simulink model "Dion_CBC_Simulink"  (R2023a)
settings: Solver=ode5  StartTime=0.0  StopTime=Inf  FixedStep=0.001  RelTol=1e-3
PostLoadFcn:
  | , if any(exist('dsrtsu_mdlpostloadfcn', 'file') ~= 0), dsrtsu_mdlpostloadfcn('Execute', bdroot); end,
InitFcn:
  | , if any(exist('rtifpga_mdlclblib', 'file') ~= 0), rtifpga_mdlclblib('Init', bdroot); end,
values from neighbouring files (symbols this model uses):
  k_harmonics = 7    [freq_sweep_continous.m]
libraries: simulink x3, rti1202lib_adc_class1 x3, rti1202lib_dac_class1 x1, rti1202lib_base x1
(part 2 of 2)

== system Dion_CBC_Simulink/invasiveness_estimator/get secondary ==
  Vector : Inport
  Demux : Demux  Outputs=[1, 1, k_harmonics-1, 1, k_harmonics-1]
  Mux : Mux  Inputs=2
  Terminator1 : Terminator
  Terminator2 : Terminator
  Terminator3 : Terminator
  secondary : Outport
  wires:
  Demux/1 -> Terminator2/1
  Mux/1 -> secondary/1
  Demux/3 -> Mux/1
  Demux/5 -> Mux/2
  Vector/1 -> Demux/1
  Demux/2 -> Terminator1/1
  Demux/4 -> Terminator3/1

== system Dion_CBC_Simulink/sig_reconstructor/Harmonic Basis Gen1 ==
  fund_freq : Inport
  Cos : Trigonometry  Operator=cos
  DC : Constant
  Gain1 : Gain  Gain=2*pi
  Integrator : Integrator
  Mux : Mux  Inputs=3
  Product : Product
  Sin : Trigonometry
  harmonics_array : Constant  Value=1:k_harmonics
  harmonic_basis : Outport  OutDataTypeStr=double  SampleTime=0
  wires:
  Gain1/1 -> Sin/1, Cos/1
  Mux/1 -> harmonic_basis/1
  Integrator/1 -> Product/1
  Cos/1 -> Mux/2
  Product/1 -> Gain1/1
  Sin/1 -> Mux/3
  harmonics_array/1 -> Product/2
  fund_freq/1 -> Integrator/1
  DC/1 -> Mux/1

== system Dion_CBC_Simulink/x_reconstructor/Harmonic Basis Gen1 ==
  fund_freq : Inport
  Cos : Trigonometry  Operator=cos
  DC : Constant
  Gain1 : Gain  Gain=2*pi
  Integrator : Integrator
  Mux : Mux  Inputs=3
  Product : Product
  Sin : Trigonometry
  harmonics_array : Constant  Value=1:k_harmonics
  harmonic_basis : Outport  OutDataTypeStr=double  SampleTime=0
  wires:
  Gain1/1 -> Sin/1, Cos/1
  Mux/1 -> harmonic_basis/1
  Integrator/1 -> Product/1
  Cos/1 -> Mux/2
  Product/1 -> Gain1/1
  Sin/1 -> Mux/3
  harmonics_array/1 -> Product/2
  fund_freq/1 -> Integrator/1
  DC/1 -> Mux/1

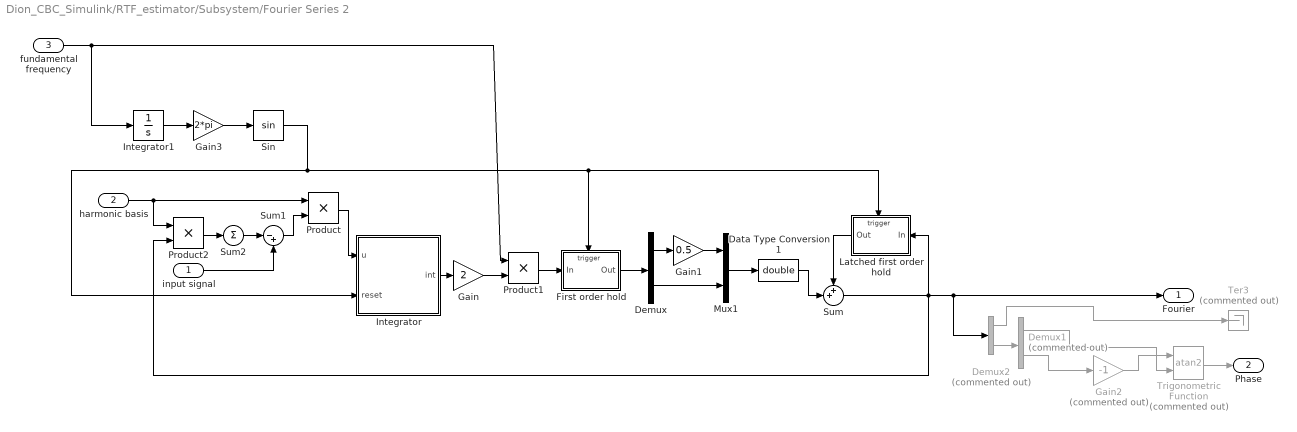
== system Dion_CBC_Simulink/RTF_estimator/Subsystem/Fourier Series 2 ==
  input signal : Inport
  harmonic basis : Inport  Port=2
  fundamental frequency : Inport  Port=3
  Data Type Conversion1 : DataTypeConversion  OutDataTypeStr=double  SaturateOnIntegerOverflow=off  RndMeth=Floor
  Demux : Demux  Outputs=[1 -1]
  Demux1 : Demux  Commented=on  Outputs=2
  Demux2 : Demux  Commented=on  Outputs=[1 -1]
  First order hold : Subsystem  TreatAsAtomicUnit=on
  Gain : Gain  Gain=2
  Gain1 : Gain  Gain=0.5
  Gain2 : Gain  Commented=on  Gain=-1
  Gain3 : Gain  Gain=2*pi
  Integrator : Subsystem
  Integrator1 : Integrator
  Latched first order hold : Subsystem  TreatAsAtomicUnit=on
  Mux1 : Mux  Inputs=2
  Product : Product  RndMeth=Zero
  Product1 : Product  RndMeth=Zero
  Product2 : Product  RndMeth=Zero
  Sin : Trigonometry
  Sum : Sum  Tag=Test  Inputs=++|
  Sum1 : Sum  Inputs=|-+
  Sum2 : Sum  Inputs=|+|
  Ter3 : Terminator  Commented=on
  Trigonometric Function : Trigonometry  Commented=on  Operator=atan2
  Fourier : Outport
  Phase : Outport  Port=2
  wires:
  fundamental frequency/1 -> Product1/1, Integrator1/1
  Integrator1/1 -> Gain3/1
  Gain3/1 -> Sin/1
  Demux2/1 -> Ter3/1
  Demux2/2 -> Demux1/1
  Gain2/1 -> Trigonometric Function/1
  Demux1/2 -> Gain2/1
  Demux1/1 -> Trigonometric Function/2
  Product/1 -> Integrator/1(u)
  Trigonometric Function/1 -> Phase/1
  Sum2/1 -> Sum1/1
  harmonic basis/1 -> Product2/1, Product/1
  input signal/1 -> Sum1/2
  Product2/1 -> Sum2/1
  Sum1/1 -> Product/2
  Latched first order hold/1(Out) -> Sum/1
  Sum/1 -> Demux2/1, Fourier/1, Latched first order hold/1(In), Product2/2
  Data Type Conversion1/1 -> Sum/2
  Mux1/1 -> Data Type Conversion1/1
  First order hold/1(Out) -> Demux/1
  Demux/2 -> Mux1/2
  Gain1/1 -> Mux1/1
  Demux/1 -> Gain1/1
  Integrator/1(int) -> Gain/1
  Sin/1 -> Latched first order hold/Trigger, First order hold/Trigger, Integrator/2(reset)
  Gain/1 -> Product1/2
  Product1/1 -> First order hold/1(In)

== system Dion_CBC_Simulink/RTF_estimator/Subsystem/Harmonic Basis Gen1 ==
  fund_freq : Inport
  Cos : Trigonometry  Operator=cos
  DC : Constant
  Gain1 : Gain  Gain=2*pi
  Integrator : Integrator
  Mux : Mux  Inputs=3
  Product : Product
  Sin : Trigonometry
  harmonics_array : Constant  Value=1:k_harmonics
  harmonic_basis : Outport  OutDataTypeStr=double  SampleTime=0
  wires:
  Gain1/1 -> Sin/1, Cos/1
  Mux/1 -> harmonic_basis/1
  Integrator/1 -> Product/1
  Cos/1 -> Mux/2
  Product/1 -> Gain1/1
  Sin/1 -> Mux/3
  harmonics_array/1 -> Product/2
  fund_freq/1 -> Integrator/1
  DC/1 -> Mux/1

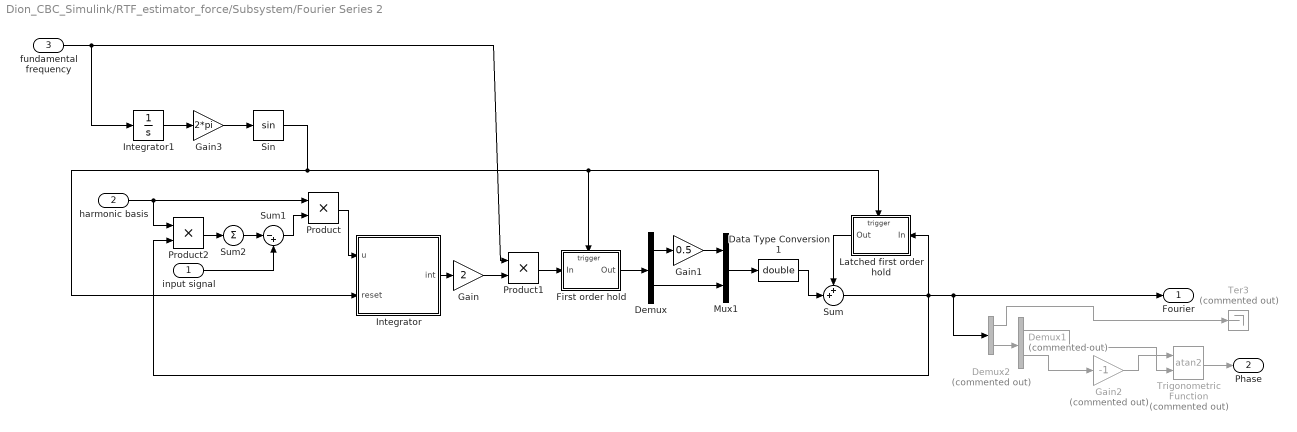
== system Dion_CBC_Simulink/RTF_estimator_force/Subsystem/Fourier Series 2 ==
  input signal : Inport
  harmonic basis : Inport  Port=2
  fundamental frequency : Inport  Port=3
  Data Type Conversion1 : DataTypeConversion  OutDataTypeStr=double  SaturateOnIntegerOverflow=off  RndMeth=Floor
  Demux : Demux  Outputs=[1 -1]
  Demux1 : Demux  Commented=on  Outputs=2
  Demux2 : Demux  Commented=on  Outputs=[1 -1]
  First order hold : Subsystem  TreatAsAtomicUnit=on
  Gain : Gain  Gain=2
  Gain1 : Gain  Gain=0.5
  Gain2 : Gain  Commented=on  Gain=-1
  Gain3 : Gain  Gain=2*pi
  Integrator : Subsystem
  Integrator1 : Integrator
  Latched first order hold : Subsystem  TreatAsAtomicUnit=on
  Mux1 : Mux  Inputs=2
  Product : Product  RndMeth=Zero
  Product1 : Product  RndMeth=Zero
  Product2 : Product  RndMeth=Zero
  Sin : Trigonometry
  Sum : Sum  Tag=Test  Inputs=++|
  Sum1 : Sum  Inputs=|-+
  Sum2 : Sum  Inputs=|+|
  Ter3 : Terminator  Commented=on
  Trigonometric Function : Trigonometry  Commented=on  Operator=atan2
  Fourier : Outport
  Phase : Outport  Port=2
  wires:
  Product1/1 -> First order hold/1(In)
  Gain/1 -> Product1/2
  Sin/1 -> Integrator/2(reset), First order hold/Trigger, Latched first order hold/Trigger
  Integrator/1(int) -> Gain/1
  Demux/1 -> Gain1/1
  Gain1/1 -> Mux1/1
  Demux/2 -> Mux1/2
  First order hold/1(Out) -> Demux/1
  Mux1/1 -> Data Type Conversion1/1
  Data Type Conversion1/1 -> Sum/2
  Sum/1 -> Product2/2, Latched first order hold/1(In), Fourier/1, Demux2/1
  Latched first order hold/1(Out) -> Sum/1
  Sum1/1 -> Product/2
  Product2/1 -> Sum2/1
  input signal/1 -> Sum1/2
  harmonic basis/1 -> Product/1, Product2/1
  Sum2/1 -> Sum1/1
  Trigonometric Function/1 -> Phase/1
  Product/1 -> Integrator/1(u)
  Demux1/1 -> Trigonometric Function/2
  Demux1/2 -> Gain2/1
  Gain2/1 -> Trigonometric Function/1
  Demux2/2 -> Demux1/1
  Demux2/1 -> Ter3/1
  Gain3/1 -> Sin/1
  Integrator1/1 -> Gain3/1
  fundamental frequency/1 -> Integrator1/1, Product1/1

== system Dion_CBC_Simulink/RTF_estimator_force/Subsystem/Harmonic Basis Gen1 ==
  fund_freq : Inport
  Cos : Trigonometry  Operator=cos
  DC : Constant
  Gain1 : Gain  Gain=2*pi
  Integrator : Integrator
  Mux : Mux  Inputs=3
  Product : Product
  Sin : Trigonometry
  harmonics_array : Constant  Value=1:k_harmonics
  harmonic_basis : Outport  OutDataTypeStr=double  SampleTime=0
  wires:
  DC/1 -> Mux/1
  fund_freq/1 -> Integrator/1
  harmonics_array/1 -> Product/2
  Sin/1 -> Mux/3
  Product/1 -> Gain1/1
  Cos/1 -> Mux/2
  Integrator/1 -> Product/1
  Mux/1 -> harmonic_basis/1
  Gain1/1 -> Cos/1, Sin/1

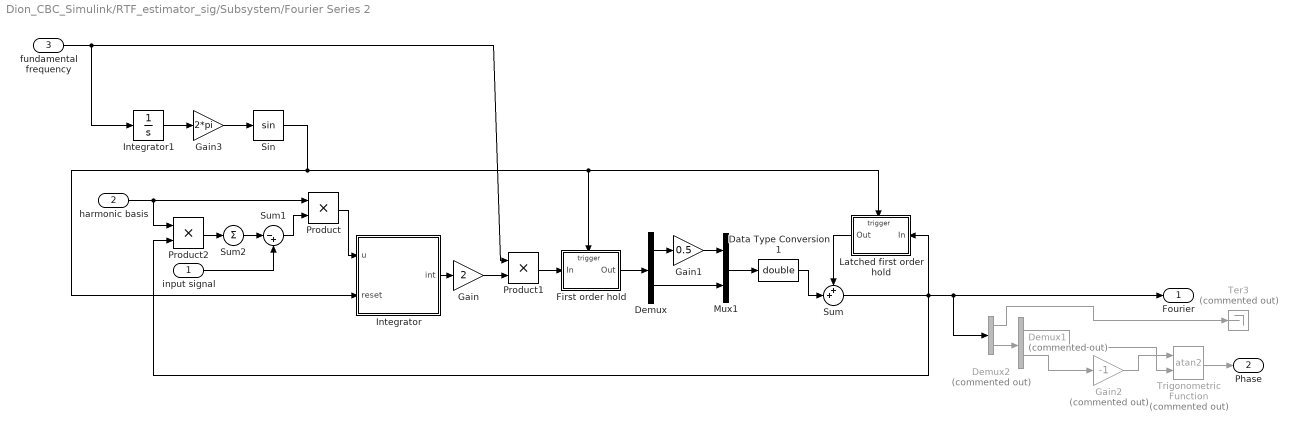
== system Dion_CBC_Simulink/RTF_estimator_sig/Subsystem/Fourier Series 2 ==
  input signal : Inport
  harmonic basis : Inport  Port=2
  fundamental frequency : Inport  Port=3
  Data Type Conversion1 : DataTypeConversion  OutDataTypeStr=double  SaturateOnIntegerOverflow=off  RndMeth=Floor
  Demux : Demux  Outputs=[1 -1]
  Demux1 : Demux  Commented=on  Outputs=2
  Demux2 : Demux  Commented=on  Outputs=[1 -1]
  First order hold : Subsystem  TreatAsAtomicUnit=on
  Gain : Gain  Gain=2
  Gain1 : Gain  Gain=0.5
  Gain2 : Gain  Commented=on  Gain=-1
  Gain3 : Gain  Gain=2*pi
  Integrator : Subsystem
  Integrator1 : Integrator
  Latched first order hold : Subsystem  TreatAsAtomicUnit=on
  Mux1 : Mux  Inputs=2
  Product : Product  RndMeth=Zero
  Product1 : Product  RndMeth=Zero
  Product2 : Product  RndMeth=Zero
  Sin : Trigonometry
  Sum : Sum  Tag=Test  Inputs=++|
  Sum1 : Sum  Inputs=|-+
  Sum2 : Sum  Inputs=|+|
  Ter3 : Terminator  Commented=on
  Trigonometric Function : Trigonometry  Commented=on  Operator=atan2
  Fourier : Outport
  Phase : Outport  Port=2
  wires:
  fundamental frequency/1 -> Product1/1, Integrator1/1
  Integrator1/1 -> Gain3/1
  Gain3/1 -> Sin/1
  Demux2/1 -> Ter3/1
  Demux2/2 -> Demux1/1
  Gain2/1 -> Trigonometric Function/1
  Demux1/2 -> Gain2/1
  Demux1/1 -> Trigonometric Function/2
  Product/1 -> Integrator/1(u)
  Trigonometric Function/1 -> Phase/1
  Sum2/1 -> Sum1/1
  harmonic basis/1 -> Product2/1, Product/1
  input signal/1 -> Sum1/2
  Product2/1 -> Sum2/1
  Sum1/1 -> Product/2
  Latched first order hold/1(Out) -> Sum/1
  Sum/1 -> Demux2/1, Fourier/1, Latched first order hold/1(In), Product2/2
  Data Type Conversion1/1 -> Sum/2
  Mux1/1 -> Data Type Conversion1/1
  First order hold/1(Out) -> Demux/1
  Demux/2 -> Mux1/2
  Gain1/1 -> Mux1/1
  Demux/1 -> Gain1/1
  Integrator/1(int) -> Gain/1
  Sin/1 -> Latched first order hold/Trigger, First order hold/Trigger, Integrator/2(reset)
  Gain/1 -> Product1/2
  Product1/1 -> First order hold/1(In)

== system Dion_CBC_Simulink/RTF_estimator_sig/Subsystem/Harmonic Basis Gen1 ==
  fund_freq : Inport
  Cos : Trigonometry  Operator=cos
  DC : Constant
  Gain1 : Gain  Gain=2*pi
  Integrator : Integrator
  Mux : Mux  Inputs=3
  Product : Product
  Sin : Trigonometry
  harmonics_array : Constant  Value=1:k_harmonics
  harmonic_basis : Outport  OutDataTypeStr=double  SampleTime=0
  wires:
  Gain1/1 -> Sin/1, Cos/1
  Mux/1 -> harmonic_basis/1
  Integrator/1 -> Product/1
  Cos/1 -> Mux/2
  Product/1 -> Gain1/1
  Sin/1 -> Mux/3
  harmonics_array/1 -> Product/2
  fund_freq/1 -> Integrator/1
  DC/1 -> Mux/1

== system Dion_CBC_Simulink/RTI Data/RTI Data Store/RTI Data Store ==
  RTI Data Store : Subsystem  mask(RTI_DATA_STORE){}
      mask help:
      | RTI Data Store Block. This block is used by RTI to store internal model dependent data. Deleting this block will result in data loss.
      |
      | NEVER DELETE, COPY, OR MODIFY THIS BLOCK!
      mask Help:
      | RTI Data Store Block. This block is used by RTI to store internal model dependent data. Deleting this block will result in data loss.
      | 
      | NEVER DELETE, COPY, OR MODIFY THIS BLOCK!
      mask Display: text(0.5, 0.5, ' ', 'HorizontalAlignment', 'center');

== system Dion_CBC_Simulink/RTF_estimator/Subsystem/Fourier Series 2/First order hold ==
  In : Inport  LatchByDelayingOutsideSignal=on
  Trigger : TriggerPort  VariantControl=(inherit)
  Out : Outport
  wires:
  In/1 -> Out/1

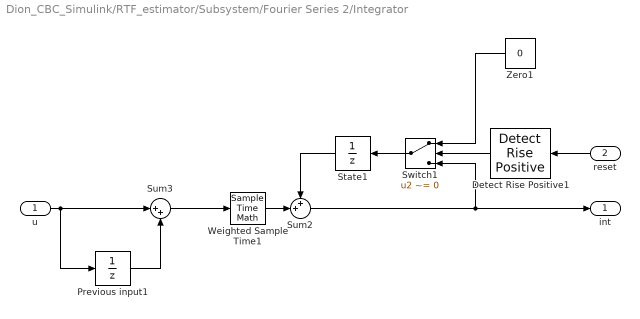
== system Dion_CBC_Simulink/RTF_estimator/Subsystem/Fourier Series 2/Integrator ==
  u : Inport
  reset : Inport  Port=2
  Detect Rise Positive1 : simulink/Logic and Bit Operations/Detect Rise Positive  vinit=0  OutDataTypeStr=uint8
  Previous input1 : UnitDelay  SampleTime=-1  HasFrameUpgradeWarning=on
  State1 : UnitDelay  SampleTime=-1  HasFrameUpgradeWarning=on
  Sum2 : Sum  Inputs=++|
  Sum3 : Sum  Inputs=|++
  Switch1 : Switch  Criteria=u2 ~= 0  SaturateOnIntegerOverflow=off  InputSameDT=off
  Weighted Sample Time1 : SampleTimeMath  TsampMathOp=*  weightValue=0.5
  Zero1 : Constant  Value=0
  int : Outport
  wires:
  State1/1 -> Sum2/1
  Sum2/1 -> Switch1/3, int/1
  Weighted Sample Time1/1 -> Sum2/2
  Sum3/1 -> Weighted Sample Time1/1
  u/1 -> Sum3/1, Previous input1/1
  Previous input1/1 -> Sum3/2
  reset/1 -> Detect Rise Positive1/1
  Switch1/1 -> State1/1
  Zero1/1 -> Switch1/1
  Detect Rise Positive1/1 -> Switch1/2

== system Dion_CBC_Simulink/RTF_estimator/Subsystem/Fourier Series 2/Latched first order hold ==
  In : Inport  LatchByDelayingOutsideSignal=on
  Trigger : TriggerPort  VariantControl=(inherit)
  Out : Outport
  wires:
  In/1 -> Out/1

== system Dion_CBC_Simulink/RTF_estimator_force/Subsystem/Fourier Series 2/First order hold ==
  In : Inport  LatchByDelayingOutsideSignal=on
  Trigger : TriggerPort  VariantControl=(inherit)
  Out : Outport
  wires:
  In/1 -> Out/1

== system Dion_CBC_Simulink/RTF_estimator_force/Subsystem/Fourier Series 2/Integrator ==
  u : Inport
  reset : Inport  Port=2
  Detect Rise Positive1 : simulink/Logic and Bit Operations/Detect Rise Positive  vinit=0  OutDataTypeStr=uint8
  Previous input1 : UnitDelay  SampleTime=-1  HasFrameUpgradeWarning=on
  State1 : UnitDelay  SampleTime=-1  HasFrameUpgradeWarning=on
  Sum2 : Sum  Inputs=++|
  Sum3 : Sum  Inputs=|++
  Switch1 : Switch  Criteria=u2 ~= 0  SaturateOnIntegerOverflow=off  InputSameDT=off
  Weighted Sample Time1 : SampleTimeMath  TsampMathOp=*  weightValue=0.5
  Zero1 : Constant  Value=0
  int : Outport
  wires:
  Detect Rise Positive1/1 -> Switch1/2
  Zero1/1 -> Switch1/1
  Switch1/1 -> State1/1
  reset/1 -> Detect Rise Positive1/1
  Previous input1/1 -> Sum3/2
  u/1 -> Previous input1/1, Sum3/1
  Sum3/1 -> Weighted Sample Time1/1
  Weighted Sample Time1/1 -> Sum2/2
  Sum2/1 -> int/1, Switch1/3
  State1/1 -> Sum2/1

== system Dion_CBC_Simulink/RTF_estimator_force/Subsystem/Fourier Series 2/Latched first order hold ==
  In : Inport  LatchByDelayingOutsideSignal=on
  Trigger : TriggerPort  VariantControl=(inherit)
  Out : Outport
  wires:
  In/1 -> Out/1

== system Dion_CBC_Simulink/RTF_estimator_sig/Subsystem/Fourier Series 2/First order hold ==
  In : Inport  LatchByDelayingOutsideSignal=on
  Trigger : TriggerPort  VariantControl=(inherit)
  Out : Outport
  wires:
  In/1 -> Out/1

== system Dion_CBC_Simulink/RTF_estimator_sig/Subsystem/Fourier Series 2/Integrator ==
  u : Inport
  reset : Inport  Port=2
  Detect Rise Positive1 : simulink/Logic and Bit Operations/Detect Rise Positive  vinit=0  OutDataTypeStr=uint8
  Previous input1 : UnitDelay  SampleTime=-1  HasFrameUpgradeWarning=on
  State1 : UnitDelay  SampleTime=-1  HasFrameUpgradeWarning=on
  Sum2 : Sum  Inputs=++|
  Sum3 : Sum  Inputs=|++
  Switch1 : Switch  Criteria=u2 ~= 0  SaturateOnIntegerOverflow=off  InputSameDT=off
  Weighted Sample Time1 : SampleTimeMath  TsampMathOp=*  weightValue=0.5
  Zero1 : Constant  Value=0
  int : Outport
  wires:
  State1/1 -> Sum2/1
  Sum2/1 -> Switch1/3, int/1
  Weighted Sample Time1/1 -> Sum2/2
  Sum3/1 -> Weighted Sample Time1/1
  u/1 -> Sum3/1, Previous input1/1
  Previous input1/1 -> Sum3/2
  reset/1 -> Detect Rise Positive1/1
  Switch1/1 -> State1/1
  Zero1/1 -> Switch1/1
  Detect Rise Positive1/1 -> Switch1/2

== system Dion_CBC_Simulink/RTF_estimator_sig/Subsystem/Fourier Series 2/Latched first order hold ==
  In : Inport  LatchByDelayingOutsideSignal=on
  Trigger : TriggerPort  VariantControl=(inherit)
  Out : Outport
  wires:
  In/1 -> Out/1

== system Dion_CBC_Simulink/RTI Data/RTI Data Store/RTI Data Store/RTI Data Store ==
  RTI Data Store : Subsystem  mask(RTI_DATA_STORE){}
      mask help:
      | RTI Data Store Block. This block is used by RTI to store internal model dependent data. Deleting this block will result in data loss.
      |
      | NEVER DELETE, COPY, OR MODIFY THIS BLOCK!
      mask Help:
      | RTI Data Store Block. This block is used by RTI to store internal model dependent data. Deleting this block will result in data loss.
      | 
      | NEVER DELETE, COPY, OR MODIFY THIS BLOCK!
      mask Display: text(0.5, 0.5, ' ', 'HorizontalAlignment', 'center');

== system Dion_CBC_Simulink/RTI Data/RTI Data Store/RTI Data Store/RTI Data Store/RTI Data Store ==

== matlab function Dion_CBC_Simulink/RTF_estimator_force/MATLAB Function1 ==
  data: Coeffs input; avgCoeffs output; varCoeffs output
function [avgCoeffs, varCoeffs] = exponentialAverageWithVariance(Coeffs)
% Exponential Moving Average (EMA) and Variance (EMV) for Fourier Coefficients

% Tuning parameter
alpha = 5e-4;  % 0.001 (slow, smooth) to 0.1 (fast, responsive)

% Persistent storage
persistent avg sqAvg
if isempty(avg)
    avg = Coeffs;
    sqAvg = Coeffs.^2;
end

% EMA update
avg = alpha * Coeffs + (1 - alpha) * avg;

% EMA of square
sqAvg = alpha * (Coeffs.^2) + (1 - alpha) * sqAvg;

% Variance = E[x^2] - (E[x])^2
varCoeffs = sqAvg - avg.^2;

% Output
avgCoeffs = avg;
end

== matlab function Dion_CBC_Simulink/RTF_estimator_sig/MATLAB Function1 ==
  data: Coeffs input; avgCoeffs output; varCoeffs output
function [avgCoeffs, varCoeffs] = exponentialAverageWithVariance(Coeffs)
% Exponential Moving Average (EMA) and Variance (EMV) for Fourier Coefficients

% Tuning parameter
alpha = 5e-4;  % 0.001 (slow, smooth) to 0.1 (fast, responsive)

% Persistent storage
persistent avg sqAvg
if isempty(avg)
    avg = Coeffs;
    sqAvg = Coeffs.^2;
end

% EMA update
avg = alpha * Coeffs + (1 - alpha) * avg;

% EMA of square
sqAvg = alpha * (Coeffs.^2) + (1 - alpha) * sqAvg;

% Variance = E[x^2] - (E[x])^2
varCoeffs = sqAvg - avg.^2;

% Output
avgCoeffs = avg;
end

== matlab function Dion_CBC_Simulink/MATLAB Function1 ==
  data: Coeffs input; avgCoeffs output; varCoeffs output
function [avgCoeffs, varCoeffs] = exponentialAverageWithVariance(Coeffs)
% Exponential Moving Average (EMA) and Variance (EMV) for Fourier Coefficients

% Tuning parameter
alpha = 5e-4;  % 0.001 (slow, smooth) to 0.1 (fast, responsive)

% Persistent storage
persistent avg sqAvg
if isempty(avg)
    avg = Coeffs;
    sqAvg = Coeffs.^2;
end

% EMA update
avg = alpha * Coeffs + (1 - alpha) * avg;

% EMA of square
sqAvg = alpha * (Coeffs.^2) + (1 - alpha) * sqAvg;

% Variance = E[x^2] - (E[x])^2
varCoeffs = sqAvg - avg.^2;

% Output
avgCoeffs = avg;
end

== matlab function Dion_CBC_Simulink/Kalman_Filter/MATLAB Function ==
  data: disp_measured input; acc_measured input; q1 input; disp_estimate output; q2 input; R input; vel_estimate output
function [disp_estimate, vel_estimate] = kalman_vel_disp(disp_measured, acc_measured, q1, q2, R)
% 雙輸入雙輸出卡爾曼觀測器，Q對角項由外部常數組裝
dt = 0.001;    % 根據你的 fs = 1000
A = [1, dt; 0, 1];
B = [0; dt];
C = [1, 0];
Q = diag([q1, q2]);
persistent xhat P inited prev_disp
if isempty(inited)
    xhat = [disp_measured; 0]; % 初值
    prev_disp = disp_measured;
    P = diag([1e-6, 100]);
    inited = true;
end
if xhat(2)==0 && prev_disp ~= disp_measured
    v0 = (disp_measured - prev_disp)/dt;
    xhat = [disp_measured; v0];
end
xhat_pred = A * xhat + B * acc_measured;
P_pred = A * P * A' + Q;
K = P_pred * C' / (C * P_pred * C' + R);
xhat = xhat_pred + K * (disp_measured - C * xhat_pred);
P = (eye(2) - K * C) * P_pred;
disp_estimate = xhat(1);
vel_estimate = xhat(2);
prev_disp = disp_measured;
end

== matlab function Dion_CBC_Simulink/RTF_estimator/MATLAB Function1 ==
  data: Coeffs input; avgCoeffs output; varCoeffs output
function [avgCoeffs, varCoeffs] = exponentialAverageWithVariance(Coeffs)
% Exponential Moving Average (EMA) and Variance (EMV) for Fourier Coefficients

% Tuning parameter
alpha = 5e-4;  % 0.001 (slow, smooth) to 0.1 (fast, responsive)

% Persistent storage
persistent avg sqAvg
if isempty(avg)
    avg = Coeffs;
    sqAvg = Coeffs.^2;
end

% EMA update
avg = alpha * Coeffs + (1 - alpha) * avg;

% EMA of square
sqAvg = alpha * (Coeffs.^2) + (1 - alpha) * sqAvg;

% Variance = E[x^2] - (E[x])^2
varCoeffs = sqAvg - avg.^2;

% Output
avgCoeffs = avg;
end
